simulink model "DisplayModel_Step1_start"  (R2013b)
settings: Solver=ode45  StartTime=0.0  StopTime=10.0  RelTol=1e-3
undefined symbols (not defined in the file): sigbuilder_block
settings Model: CovHTMLOptions=-sRT=1 -aTS=1 -bRG=1 -bTC=1 -hTR=0 -nFC=0 -scm=1 -bcm=1 -xEv=0  Creator=siddhars  LastModifiedBy=rruff
settings OptimizationCC: ExpressionDepthLimit=2147483647
settings DebuggingCC: StateNameClashWarn=warning

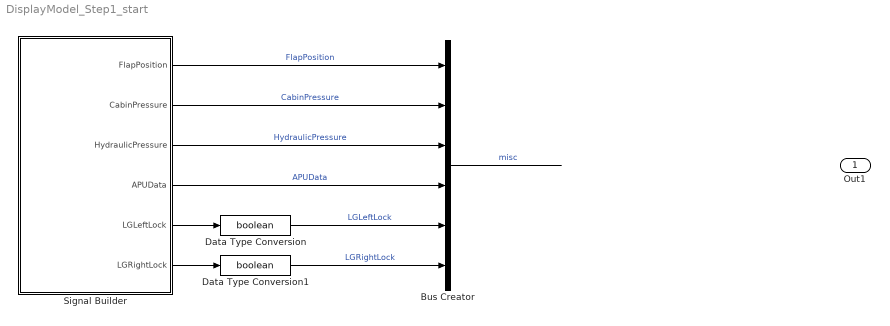
== system DisplayModel_Step1_start ==
  Bus Creator : BusCreator  Inputs=6  OutDataTypeStr=Bus: MiscData
  Data Type Conversion : DataTypeConversion  OutDataTypeStr=boolean
  Data Type Conversion1 : DataTypeConversion  OutDataTypeStr=boolean
  Signal Builder : Subsystem  Tag=STV Subsys  LoadFcn=sigbuilder_block('load');  StartFcn=sigbuilder_block('start');  StopFcn=sigbuilder_block('stop');  ClipboardFcn=sigbuilder_block('clipboard');  mask(Sigbuilder block){}
      mask help: Simulink:masks:SigbuilderBlock_MD
      mask init:
      | if ~strcmp(get_param(bdroot(gcbh),'SimulationStatus'),'stopped') tuvar = sigbuilder_block('maskInit'); end
      settings: CopyFcn=sigbuilder_block('copy');  DeleteFcn=sigbuilder_block('delete');  ModelCloseFcn=sigbuilder_block('modelClose');  PreSaveFcn=sigbuilder_block('preSave');  PauseFcn=sigbuilder_block('pause');  ContinueFcn=sigbuilder_block('continue');  NameChangeFcn=sigbuilder_block('namechange');  OpenFcn=sigbuilder_block('open',[43.5 185.25 692.25 402.75 ]);  CloseFcn=sigbuilder_block('close');
      mask Display: plot(0, 0, 100, 100,[2, 2, 32, 32, 2], [68, 8, 8, 68, 68],[32, 2], [38, 38], [32, 19, 2],[53, 60, 44], [32, 17, 17, 2],[16, 16, 31, 31]);txt = getActiveGroup(gcbh);text(2, 100, txt,'verticalAlignment', 'top');
  Out1 : Outport
  wires:
  Signal Builder/6(LGRightLock) -> Data Type Conversion1/1
  Signal Builder/5(LGLeftLock) -> Data Type Conversion/1
  Data Type Conversion1/1 -> Bus Creator/6  "LGRightLock"
  Data Type Conversion/1 -> Bus Creator/5  "LGLeftLock"
  ? -> Out1/1
  Signal Builder/1(FlapPosition) -> Bus Creator/1  "FlapPosition"
  Signal Builder/3(HydraulicPressure) -> Bus Creator/3  "HydraulicPressure"
  Signal Builder/4(APUData) -> Bus Creator/4  "APUData"
  Signal Builder/2(CabinPressure) -> Bus Creator/2  "CabinPressure"
  Bus Creator/1 -> ?  "misc"

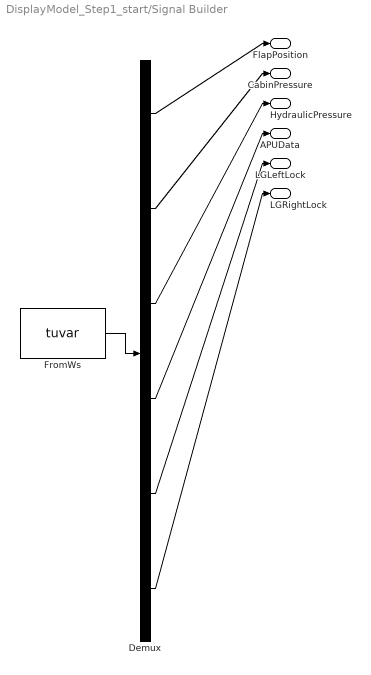
== system DisplayModel_Step1_start/Signal Builder ==
  Demux : Demux  Tag=STV Demux  Outputs=6
  FromWs : FromWorkspace  Tag=STV FromWs  VariableName=tuvar  SampleTime=0
      SigBuilderData=|
      | common.afterFinalStr = 'Extrapolate'
      | common.sampleTime = 0
      | dataSet(1).timeRange = [0 10]
      | dataSet(1).name = 'BothOn'
      | dataSet(2).timeRange = [0 10]
      | dataSet(2).name = 'OneOnA'
      | dataSet(3).timeRange = [0 10]
      | dataSet(3).name = 'OneOnB'
      | dataSet(4).timeRange = [0 10]
      | dataSet(4).name = 'BothOFF'
      | sbobj.Groups(1).Name = 'BothOn'
      | sbobj.Groups(1).Signals(1).Name = 'FlapPosition'
      | sbobj.Groups(1).Signals(1).XData = [0 10]
      | sbobj.Groups(1).Signals(1).YData = [0 0]
      | sbobj.Groups(1).Signals(2).Name = 'CabinPressure'
      | sbobj.Groups(1).Signals(2).XData = [0 10]
      | sbobj.Groups(1).Signals(2).YData = [0 0]
      | sbobj.Groups(1).Signals(3).Name = 'HydraulicPressure'
      | sbobj.Groups(1).Signals(3).XData = [0 10]
      | sbobj.Groups(1).Signals(3).YData = [0 0]
      | sbobj.Groups(1).Signals(4).Name = 'APUData'
      | sbobj.Groups(1).Signals(4).XData = [0 10]
      | sbobj.Groups(1).Signals(4).YData = [0 0]
      | sbobj.Groups(1).Signals(5).Name = 'LGLeftLock'
      | sbobj.Groups(1).Signals(5).XData = [0 1.74 6.62 10]
      | sbobj.Groups(1).Signals(5).YData = [1 1 1 1]
      | sbobj.Groups(1).Signals(6).Name = 'LGRightLock'
      | sbobj.Groups(1).Signals(6).XData = [0 3.36 7.8 10]
      | sbobj.Groups(1).Signals(6).YData = [1 1 1 1]
      | sbobj.Groups(2).Name = 'OneOnA'
      | sbobj.Groups(2).Signals(1).Name = 'FlapPosition'
      | sbobj.Groups(2).Signals(1).XData = [0 10]
      | sbobj.Groups(2).Signals(1).YData = [0 0]
      | sbobj.Groups(2).Signals(2).Name = 'CabinPressure'
      | sbobj.Groups(2).Signals(2).XData = [0 10]
      | sbobj.Groups(2).Signals(2).YData = [0 0]
      | sbobj.Groups(2).Signals(3).Name = 'HydraulicPressure'
      | sbobj.Groups(2).Signals(3).XData = [0 10]
      | sbobj.Groups(2).Signals(3).YData = [0 0]
      | sbobj.Groups(2).Signals(4).Name = 'APUData'
      | sbobj.Groups(2).Signals(4).XData = [0 10]
      | sbobj.Groups(2).Signals(4).YData = [0 0]
      | sbobj.Groups(2).Signals(5).Name = 'LGLeftLock'
      | sbobj.Groups(2).Signals(5).XData = [0 5.02 5.02 10]
      | sbobj.Groups(2).Signals(5).YData = [1 1 0 0]
      | sbobj.Groups(2).Signals(6).Name = 'LGRightLock'
      | sbobj.Groups(2).Signals(6).XData = [0 5.02 5.02 10]
      | sbobj.Groups(2).Signals(6).YData = [0 0 1 1]
      | sbobj.Groups(3).Name = 'OneOnB'
      | sbobj.Groups(3).Signals(1).Name = 'FlapPosition'
      | sbobj.Groups(3).Signals(1).XData = [0 10]
      | sbobj.Groups(3).Signals(1).YData = [0 0]
      | sbobj.Groups(3).Signals(2).Name = 'CabinPressure'
      | sbobj.Groups(3).Signals(2).XData = [0 10]
      | sbobj.Groups(3).Signals(2).YData = [0 0]
      | sbobj.Groups(3).Signals(3).Name = 'HydraulicPressure'
      | sbobj.Groups(3).Signals(3).XData = [0 10]
      | sbobj.Groups(3).Signals(3).YData = [0 0]
      | sbobj.Groups(3).Signals(4).Name = 'APUData'
      | sbobj.Groups(3).Signals(4).XData = [0 10]
      | sbobj.Groups(3).Signals(4).YData = [0 0]
      | sbobj.Groups(3).Signals(5).Name = 'LGLeftLock'
      | sbobj.Groups(3).Signals(5).XData = [0 5.02 5.02 10]
      | sbobj.Groups(3).Signals(5).YData = [0 0 1 1]
      | sbobj.Groups(3).Signals(6).Name = 'LGRightLock'
      | sbobj.Groups(3).Signals(6).XData = [0 5.02 5.02 10]
      | sbobj.Groups(3).Signals(6).YData = [1 1 0 0]
      | sbobj.Groups(4).Name = 'BothOFF'
      | sbobj.Groups(4).Signals(1).Name = 'FlapPosition'
      | sbobj.Groups(4).Signals(1).XData = [0 10]
      | sbobj.Groups(4).Signals(1).YData = [0 0]
      | sbobj.Groups(4).Signals(2).Name = 'CabinPressure'
      | sbobj.Groups(4).Signals(2).XData = [0 10]
      | sbobj.Groups(4).Signals(2).YData = [0 0]
      | sbobj.Groups(4).Signals(3).Name = 'HydraulicPressure'
      | sbobj.Groups(4).Signals(3).XData = [0 10]
      | sbobj.Groups(4).Signals(3).YData = [0 0]
      | sbobj.Groups(4).Signals(4).Name = 'APUData'
      | sbobj.Groups(4).Signals(4).XData = [0 10]
      | sbobj.Groups(4).Signals(4).YData = [0 0]
      | sbobj.Groups(4).Signals(5).Name = 'LGLeftLock'
      | sbobj.Groups(4).Signals(5).XData = [0 10]
      | sbobj.Groups(4).Signals(5).YData = [0 0]
      | sbobj.Groups(4).Signals(6).Name = 'LGRightLock'
      | sbobj.Groups(4).Signals(6).XData = [0 10]
      | sbobj.Groups(4).Signals(6).YData = [0 0]
  FlapPosition : Outport  Tag=STV Outport
  CabinPressure : Outport  Tag=STV Outport  Port=2
  HydraulicPressure : Outport  Tag=STV Outport  Port=3
  APUData : Outport  Tag=STV Outport  Port=4
  LGLeftLock : Outport  Tag=STV Outport  Port=5
  LGRightLock : Outport  Tag=STV Outport  Port=6
  wires:
  FromWs/1 -> Demux/1
  Demux/1 -> FlapPosition/1
  Demux/2 -> CabinPressure/1
  Demux/3 -> HydraulicPressure/1
  Demux/4 -> APUData/1
  Demux/5 -> LGLeftLock/1
  Demux/6 -> LGRightLock/1
